simulink model "monitoring3_TP511_student_filtrace_determine_b"  (R2013a)
settings: Solver=ode4  StartTime=0.0  StopTime=timing  FixedStep=0.0001  RelTol=1e-3
values from neighbouring files (symbols this model uses):
  timing = round(timing*0.8)    [run_simulations_and_create_graphs.m]
  w = i    [run_simulations_and_create_graphs.m]
undefined symbols (not defined in the file or in its folder): Humusoft, MF634
libraries: rtwinlib x5, dsparch4 x2, simulink x2
settings Model: Creator=kat352  LastModifiedBy=kat352
settings DebuggingCC: FcnCallInpInsideContextMsg=EnableAllAsWarning
settings HardwareCC: ProdBitPerInt=16  ProdBitPerPointer=16  ProdWordSize=16  ProdHWDeviceType=Generic->16-bit Embedded Processor
settings RTWCC: SystemTargetFile=rtwin.tlc  TemplateMakefile=rtwin.tmf  Description=Real-Time Windows Target  ProcessScript=rtwin_make_rtw_hook  RTWCompilerOptimization=On
settings CodeAppCC: MaxIdLength=95
settings TargetCC: TargetLibSuffix=_rtwin.lib  TargetPreCompLibLocation=C:\Program Files\MATLAB\R2013a\toolbox\rtw\targets\rtwin\lib\win64  CodeReplacementLibrary=ANSI_C  IsPILTarget=off  EnableShiftOperators=on

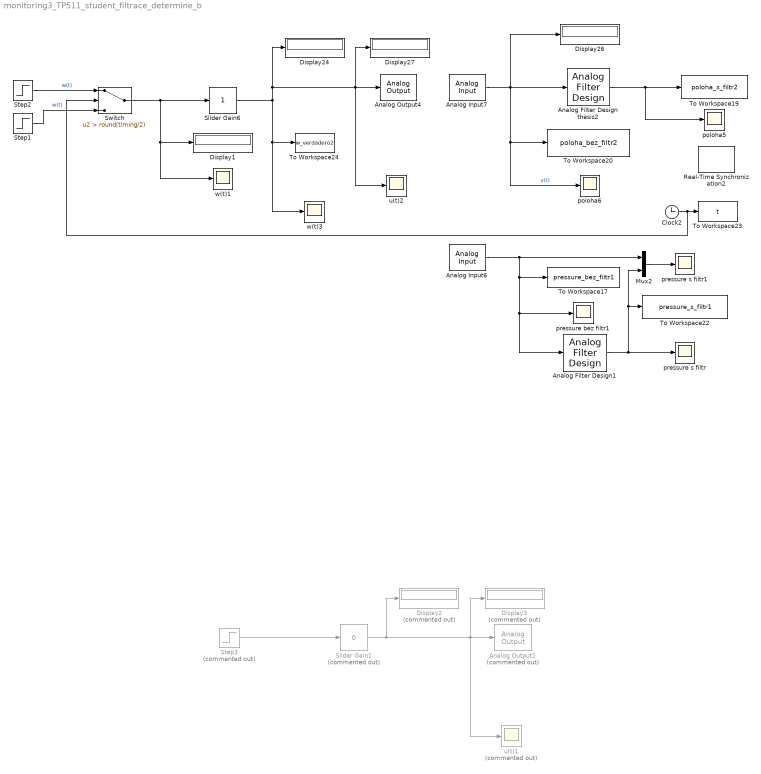
== system monitoring3_TP511_student_filtrace_determine_b ==
  Analog Filter Design thesis2 : dsparch4/Analog Filter Design  method=Butterworth  filttype=Lowpass  N=1  Wlo=300  Whi=80  Rp=2  Rs=40
  Analog Filter Design1 : dsparch4/Analog Filter Design  method=Butterworth  filttype=Lowpass  N=1  Wlo=300  Whi=80  Rp=2  Rs=40
  Analog Input6 : rtwinlib/Analog Input  SampleTime=-1  MaxMissedTicks=10000  ShowMissedTicks=off  YieldWhenWaiting=off  DrvName=Humusoft/MF634  DrvAddress=4294967295  DrvOptions=0  Channels=2  RangeMode=1  VoltRange=1  DataType=1
      settings: AttributesFormatString=Humusoft\nMF634 [auto]
  Analog Input7 : rtwinlib/Analog Input  SampleTime=-1  MaxMissedTicks=10000  ShowMissedTicks=off  YieldWhenWaiting=off  DrvName=Humusoft/MF634  DrvAddress=4294967295  DrvOptions=0  Channels=1  RangeMode=1  VoltRange=1  DataType=1
      settings: AttributesFormatString=Humusoft\nMF634 [auto]
  Analog Output1 : rtwinlib/Analog Output  Commented=on  SampleTime=-1  MaxMissedTicks=10000  ShowMissedTicks=off  YieldWhenWaiting=off  DrvName=Humusoft/MF634  DrvAddress=4294967295  DrvOptions=0  Channels=1  RangeMode=1  VoltRange=1  InitialValue=[]  FinalValue=[]
      settings: AttributesFormatString=Humusoft\nMF634 [auto]
  Analog Output4 : rtwinlib/Analog Output  SampleTime=-1  MaxMissedTicks=10000  ShowMissedTicks=off  YieldWhenWaiting=off  DrvName=Humusoft/MF634  DrvAddress=4294967295  DrvOptions=0  Channels=1  RangeMode=1  VoltRange=1  InitialValue=[]  FinalValue=[]
      settings: AttributesFormatString=Humusoft\nMF634 [auto]
  Clock2 : Clock
  Display{1,24,26..27} (4 alike) : Display
  Display2 : Display  Commented=on
  Display3 : Display  Commented=on
  Mux2 : Mux  Inputs=2
  Real-Time Synchronization2 : rtwinlib/Real-Time Synchronization  SampleTime=-1  MaxMissedTicks=100000  ShowMissedTicks=off  YieldWhenWaiting=off
  Slider Gain1 : simulink/Math Operations/Slider Gain  Commented=on  low=-10  gain=0  high=10
  Slider Gain6 : simulink/Math Operations/Slider Gain  low=-10  gain=1  high=10
  Step1 : Step  Time=0.1  After=w  SampleTime=0
  Step2 : Step  Time=round(timing/2) + 0.1  After=-w  SampleTime=0
  Step3 : Step  Commented=on  Time=0.1  After=2  SampleTime=0
  Switch : Switch  Criteria=u2 > Threshold  Threshold=round(timing/2)
  To Workspace17 : ToWorkspace  VariableName=pressure_bez_filtr1  SampleTime=-1
  To Workspace19 : ToWorkspace  VariableName=poloha_s_filtr2  SampleTime=-1
  To Workspace20 : ToWorkspace  VariableName=poloha_bez_filtr2  SampleTime=-1
  To Workspace22 : ToWorkspace  VariableName=pressure_s_filtr1  SampleTime=-1
  To Workspace23 : ToWorkspace  VariableName=t  SampleTime=-1
  To Workspace24 : ToWorkspace  VariableName=w_verdadero2  SampleTime=-1
  poloha5 : Scope
      settings: TimeRange=6  YMin=0  YMax=0.2  SaveName=ScopeData22  MaxDataPoints=50000000
  poloha6 : Scope
      settings: TimeRange=50  YMin=6.75  YMax=8.75  SaveName=ScopeData23  MaxDataPoints=50000000
  pressure bez filtr1 : Scope
      settings: TimeRange=25  YMin=-10  YMax=0.5  SaveName=ScopeData24  MaxDataPoints=50000000
  pressure s filtr : Scope
      settings: TimeRange=25  YMin=5.94  YMax=5.98  SaveName=ScopeData28  MaxDataPoints=50000000
  pressure s filtr1 : Scope
      settings: TimeRange=25  YMin=-10.5  YMax=0.5  SaveName=ScopeData25  MaxDataPoints=50000000
  u(t)1 : Scope  Commented=on
      settings: TimeRange=6  YMin=-10  YMax=0  MaxDataPoints=50000000
  u(t)2 : Scope
      settings: TimeRange=6  YMin=-10  YMax=0  SaveName=ScopeData26  MaxDataPoints=50000000
  w(t)1 : Scope
      settings: TimeRange=6  YMin=-4  YMax=0  MaxDataPoints=50000000
  w(t)3 : Scope
      settings: TimeRange=6  YMin=-4  YMax=0  SaveName=ScopeData27  MaxDataPoints=50000000
  wires:
  Analog Input6/1 -> Analog Filter Design1/1, pressure bez filtr1/1, To Workspace17/1, Mux2/1
  Analog Filter Design thesis2/1 -> poloha5/1, To Workspace19/1
  Analog Filter Design1/1 -> Mux2/2, To Workspace22/1, pressure s filtr/1
  Mux2/1 -> pressure s filtr1/1
  Clock2/1 -> Switch/2, To Workspace23/1
  Slider Gain6/1 -> Display24/1, Display27/1, u(t)2/1, Analog Output4/1, To Workspace24/1, w(t)3/1
  Analog Input7/1 -> Display26/1, Analog Filter Design thesis2/1, poloha6/1, To Workspace20/1  "y(t)"
  Switch/1 -> w(t)1/1, Display1/1, Slider Gain6/1
  Step2/1 -> Switch/1  "w(t)"
  Step1/1 -> Switch/3  "w(t)"
  Slider Gain1/1 -> Display2/1, Display3/1, u(t)1/1, Analog Output1/1
  Step3/1 -> Slider Gain1/1
